simulink model "p1"  (R2015a)
settings: Solver=ode45  StartTime=0.0  StopTime=100  FixedStep=0.1  RelTol=1e-8
libraries: simulink x1
settings Model: Creator=vdrouinv  LastModifiedBy=vdrouinv

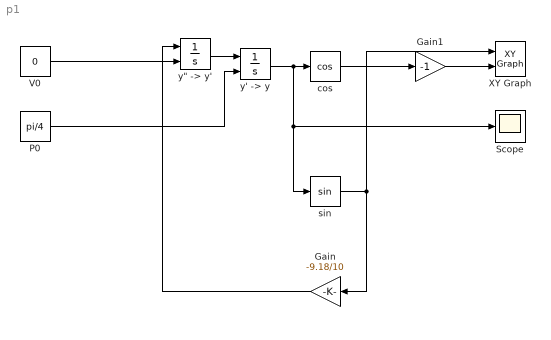
== system p1 ==
  Gain : Gain  Gain=-9.18/10
  Gain1 : Gain  Gain=-1
  P0 : Constant  Value=pi/4
  Scope : Scope
  V0 : Constant  Value=0
  XY Graph : simulink/Sinks/XY Graph  xmin=-1  xmax=1  ymin=-1  ymax=1  st=-1
  cos : Trigonometry  Operator=cos
  sin : Trigonometry
  "y\" -> y'" : Integrator  InitialConditionSource=external
  "y' -> y" : Integrator  InitialConditionSource=external
  wires:
  sin/1 -> XY Graph/1, Gain/1
  "y\" -> y'"/1 -> "y' -> y"/1
  "y' -> y"/1 -> sin/1, Scope/1, cos/1
  Gain/1 -> "y\" -> y'"/1
  P0/1 -> "y' -> y"/2
  V0/1 -> "y\" -> y'"/2
  cos/1 -> Gain1/1
  Gain1/1 -> XY Graph/2
